simulink model "Estimator_Model_tune"  (R2017b)
settings: Solver=FixedStepAuto  StartTime=0.0  StopTime=T  FixedStep=0.01  RelTol=1e-3
values from neighbouring files (symbols this model uses):
  Cf = 80000    [Init_for_washout_filter.m]
  Cr = 85000    [Init_for_washout_filter.m]
  L = lf+lr    (= 2.55)    [Init_for_washout_filter.m]
  lf = 0.41*2.55    (= 1.0455)    [Init_for_washout_filter.m]
  lr = 2.55-lf    (= 1.5045)    [Init_for_washout_filter.m]
  mass = 1435-80    (= 1355)    [Init_for_washout_filter.m]
  rollGrad = 5*(pi/180)    (= 0.0872664625997)    [Init_for_washout_filter.m]
  T_w = i*0.5    [mainscript.m]
settings Model: Creator=gandh  LastModifiedBy=Dell

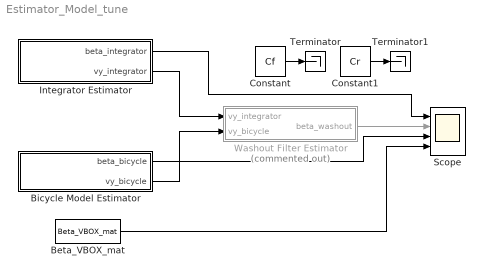
== system Estimator_Model_tune ==
  Beta_VBOX_mat : FromWorkspace  VariableName=Beta_VBOX_mat  SampleTime=0
  Bicycle Model Estimator : Subsystem
  Constant : Constant  Value=Cf
  Constant1 : Constant  Value=Cr
  Integrator Estimator : Subsystem
  Scope : Scope  NumInputPorts=4
  Terminator : Terminator
  Terminator1 : Terminator
  Washout Filter Estimator : Subsystem  Commented=on
  wires:
  Integrator Estimator/1(beta_integrator) -> Scope/1
  Integrator Estimator/2("vy_integrator ") -> Washout Filter Estimator/1(vy_integrator)
  Bicycle Model Estimator/2(vy_bicycle) -> Washout Filter Estimator/2(vy_bicycle)
  Beta_VBOX_mat/1 -> Scope/4
  Bicycle Model Estimator/1(beta_bicycle) -> Scope/3
  Washout Filter Estimator/1(beta_washout) -> Scope/2
  Constant/1 -> Terminator/1
  Constant1/1 -> Terminator1/1

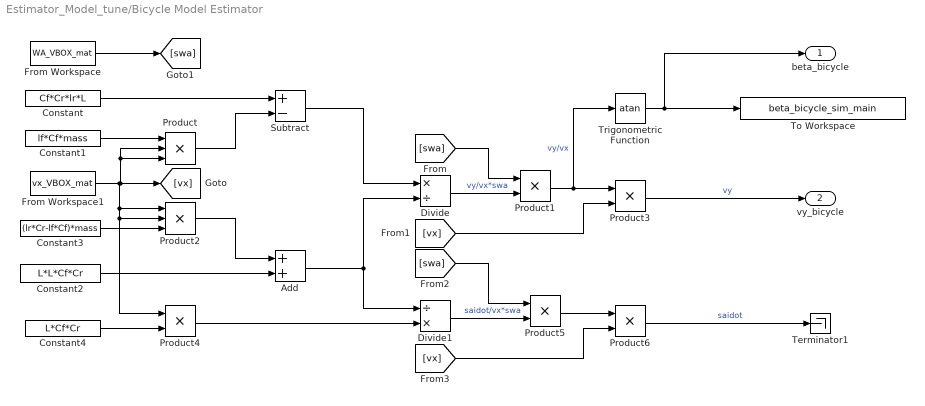
== system Estimator_Model_tune/Bicycle Model Estimator ==
  Add : Sum
  Constant : Constant  Value=Cf*Cr*lr*L
  Constant1 : Constant  Value=lf*Cf*mass
  Constant2 : Constant  Value=L*L*Cf*Cr
  Constant3 : Constant  Value=(lr*Cr-lf*Cf)*mass
  Constant4 : Constant  Value=L*Cf*Cr
  Divide : Product  Inputs=*/
  Divide1 : Product  Inputs=/*
  From Workspace : FromWorkspace  VariableName=WA_VBOX_mat  SampleTime=0
  From Workspace1 : FromWorkspace  VariableName=vx_VBOX_mat  SampleTime=0
  Product : Product  Inputs=3
  Product{1,3..6} (5 alike) : Product
  Product2 : Product  Inputs=3
  Subtract : Sum  Inputs=+-
  Terminator1 : Terminator
  To Workspace : ToWorkspace  VariableName=beta_bicycle_sim_main  SaveFormat=Timeseries  SampleTime=-1
  Trigonometric Function : Trigonometry  Operator=atan
  beta_bicycle : Outport
  vy_bicycle : Outport  Port=2
  wires:
  [vx] -> Product3/2
  Constant2/1 -> Add/2
  Product1/1 -> Trigonometric Function/1, Product3/1  "vy/vx"
  Add/1 -> Divide1/1, Divide/2
  Trigonometric Function/1 -> beta_bicycle/1, To Workspace/1
  Constant/1 -> Subtract/1
  Product3/1 -> vy_bicycle/1  "vy"
  Divide1/1 -> Product5/2  "saidot/vx*swa"
  [swa] -> Product1/1
  From Workspace1/1 -> Product2/2, Product4/1, Product2/1, [vx], Product/3, Product/2
  Product6/1 -> Terminator1/1  "saidot"
  Constant1/1 -> Product/1
  Constant4/1 -> Product4/2
  From Workspace/1 -> [swa]
  Divide/1 -> Product1/2  "vy/vx*swa"
  Product/1 -> Subtract/2
  Constant3/1 -> Product2/3
  Product5/1 -> Product6/1
  Product2/1 -> Add/1
  Subtract/1 -> Divide/1
  [vx] -> Product6/2
  [swa] -> Product5/1
  Product4/1 -> Divide1/2

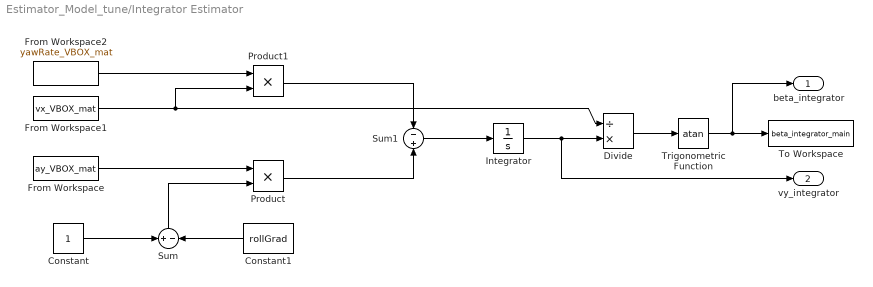
== system Estimator_Model_tune/Integrator Estimator ==
  Constant : Constant
  Constant1 : Constant  Value=rollGrad
  Divide : Product  Inputs=/*
  From Workspace : FromWorkspace  VariableName=ay_VBOX_mat  SampleTime=0
  From Workspace1 : FromWorkspace  VariableName=vx_VBOX_mat  SampleTime=0
  From Workspace2 : FromWorkspace  VariableName=yawRate_VBOX_mat  SampleTime=0
  Integrator : Integrator
  Product : Product
  Product1 : Product
  Sum : Sum  Inputs=+-
  Sum1 : Sum  Inputs=-+
  To Workspace : ToWorkspace  VariableName=beta_integrator_main  SaveFormat=Timeseries  SampleTime=-1
  Trigonometric Function : Trigonometry  Operator=atan
  beta_integrator : Outport
  "vy_integrator " : Outport  Port=2
  wires:
  Trigonometric Function/1 -> beta_integrator/1, To Workspace/1
  From Workspace/1 -> Product/1
  From Workspace1/1 -> Divide/1, Product1/2
  Constant/1 -> Sum/1
  Product/1 -> Sum1/2
  Constant1/1 -> Sum/2
  From Workspace2/1 -> Product1/1
  Product1/1 -> Sum1/1
  Divide/1 -> Trigonometric Function/1
  Sum1/1 -> Integrator/1
  Sum/1 -> Product/2
  Integrator/1 -> "vy_integrator "/1, Divide/2

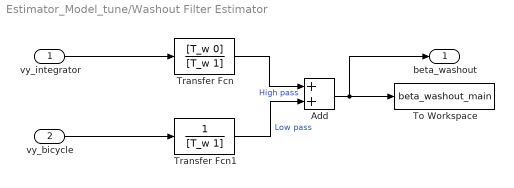
== system Estimator_Model_tune/Washout Filter Estimator ==
  vy_integrator : Inport
  vy_bicycle : Inport  Port=2
  Add : Sum
  To Workspace : ToWorkspace  VariableName=beta_washout_main  SaveFormat=Timeseries  SampleTime=-1
  Transfer Fcn : TransferFcn  Numerator=[T_w 0]  Denominator=[T_w 1]
  Transfer Fcn1 : TransferFcn  Denominator=[T_w 1]
  beta_washout : Outport
  wires:
  vy_integrator/1 -> Transfer Fcn/1
  Add/1 -> beta_washout/1, To Workspace/1
  Transfer Fcn1/1 -> Add/2  "Low pass"
  vy_bicycle/1 -> Transfer Fcn1/1
  Transfer Fcn/1 -> Add/1  "High pass"
